simulink subsystem "Controller"  (R2020a)
settings: Solver=VariableStepAuto  StartTime=0.0  StopTime=10.0  RelTol=1e-3
values from neighbouring files (symbols this model uses):
  TMAX = { 32; 32; 32; 32; 32; 32; 32; 32}    [main_adaptive_mpc.m]    (also in matlab.mat = [32 32 32 32 32 32 32 32])
  TMIN = {-26;-26;-26;-26;-26;-26;-26;-26}    [main_adaptive_mpc.m]    (also in matlab.mat = [-26 -26 -26 -26 -26 -26 -26 -26])
  Ts = 0.1    [main_adaptive_mpc.m]    (also in matlab.mat; newNewTraj.m = 0.25; plant_init.m)
  Ui = zeros(1,nU)    [GetAuvSimAndJacobian.m]    (also in main_adaptive_mpc.m = [0;0;0;0;0;0;0;0]; matlab.mat = [0 0 0 0 0 0 0 0])
  Xi = zeros(1,nX)    [GetAuvSimAndJacobian.m]    (also in main_adaptive_mpc.m = [0;0;0;0;0;0;0;0;0;0;0;0]; matlab.mat = [0 0 0 1 0 0 0 0 0 0 0 0 ... (13 elements, 13x1)])
libraries: mpclib x1
settings Model: Creator=Lamarre  LastModifiedBy=Lamarre

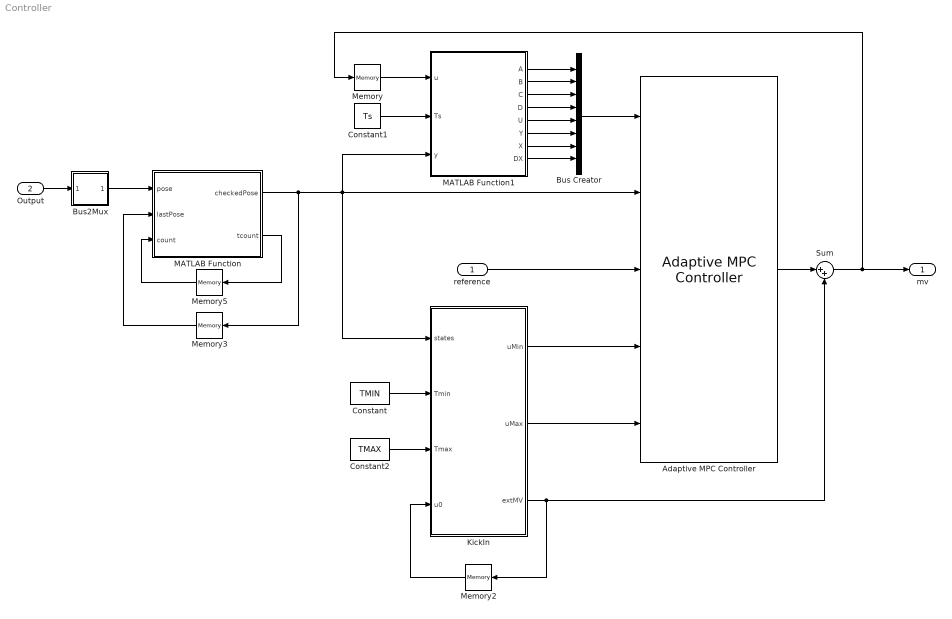
== system Controller ==
  reference : Inport
  Output : Inport  Port=2
  Adaptive MPC Controller : mpclib/Adaptive MPC Controller  SCDEnableBlockLinearizationSpecification=on  mpcobj=mpcobj  enable_value=0  updateMPCinCallerWorkspace=on  md_inport=off  mv_inport=off  uref_inport=off  return_cost=off  return_mvseq=off  return_qpstatus=off  return_xseq=off  return_state=off  return_ovseq=off  state_inport=off  isltv_plant=off  umin_inport=on  umax_inport=on  ymin_inport=off  ymax_inport=off  cc_inport=off  ywt_inport=off  uwt_inport=off  duwt_inport=off  rhoeps_inport=off  pm_inport=off  MaximumP=10  HorizonChoice=FixedHorizon  BlockDataType=double  SampleTimeInherited=off  switch_inport=off
  Bus Creator : BusCreator  Inputs=8
  Bus2Mux : Subsystem
  Constant : Constant  Value=TMIN  VectorParams1D=off
  Constant1 : Constant  Value=Ts
  Constant2 : Constant  Value=TMAX
  KickIn : MATLAB Function  TreatAsAtomicUnit=on  SystemSampleTime=Ts
  MATLAB Function : MATLAB Function  TreatAsAtomicUnit=on
  MATLAB Function1 : MATLAB Function  TreatAsAtomicUnit=on  SystemSampleTime=Ts
  Memory : Memory  InitialCondition=Ui
  Memory2 : Memory  InitialCondition=[0;0;0;0;-7.1;6.94;-7.49;7.65]
  Memory3 : Memory  InitialCondition=Xi
  Memory5 : Memory  InitialCondition=[0,0,0]
  Sum : Sum  Inputs=|++
  mv : Outport
  wires:
  Sum/1 -> mv/1, Memory/1
  Adaptive MPC Controller/1 -> Sum/1
  MATLAB Function1/2(B) -> Bus Creator/2
  MATLAB Function1/1(A) -> Bus Creator/1
  MATLAB Function1/6(Y) -> Bus Creator/6
  MATLAB Function1/8(DX) -> Bus Creator/8
  MATLAB Function1/3(C) -> Bus Creator/3
  MATLAB Function1/4(D) -> Bus Creator/4
  MATLAB Function1/5(U) -> Bus Creator/5
  MATLAB Function1/7(X) -> Bus Creator/7
  Bus Creator/1 -> Adaptive MPC Controller/1
  Memory/1 -> MATLAB Function1/1(u)
  Constant1/1 -> MATLAB Function1/2(Ts)
  KickIn/3(extMV) -> Memory2/1, Sum/2
  Constant2/1 -> KickIn/3(Tmax)
  Memory2/1 -> KickIn/4(u0)
  Constant/1 -> KickIn/2(Tmin)
  KickIn/1(uMin) -> Adaptive MPC Controller/4
  KickIn/2(uMax) -> Adaptive MPC Controller/5
  Output/1 -> Bus2Mux/1(In1)
  Memory5/1 -> MATLAB Function/3(count)
  Memory3/1 -> MATLAB Function/2(lastPose)
  Bus2Mux/1(Out1) -> MATLAB Function/1(pose)
  MATLAB Function/2(tcount) -> Memory5/1
  MATLAB Function/1(checkedPose) -> Memory3/1, MATLAB Function1/3(y), Adaptive MPC Controller/2, KickIn/1(states)
  reference/1 -> Adaptive MPC Controller/3

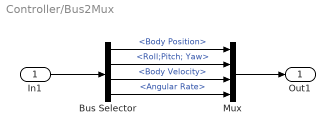
== system Controller/Bus2Mux ==
  In1 : Inport
  Bus Selector : BusSelector  OutputSignals=Body Position,Roll;Pitch; Yaw,Body Velocity,Angular Rate
  Mux : Mux
  Out1 : Outport
  wires:
  Mux/1 -> Out1/1
  In1/1 -> Bus Selector/1
  Bus Selector/2 -> Mux/2  "<Roll;Pitch; Yaw>"
  Bus Selector/4 -> Mux/4  "<Angular Rate>"
  Bus Selector/1 -> Mux/1  "<Body Position>"
  Bus Selector/3 -> Mux/3  "<Body Velocity>"

== matlab function Controller/MATLAB Function1 ==
  data: u input; Ts input; y input; A output; B output; C output; D output; U output; Y output; X output; DX output
function [A,B,C,D,U,Y,X,DX] = TrimPlant(u,Ts,y)
% Lineariser le model dynamique

%x=[y(4:5,1);y(7:12,1)];
%x(5)=x(5)-.85;
[Ac, Bc, Cc, Dc]=AUVStateJacobianFcn(y,u);
% Generate discrete-time model

%  nx = size(Ac,1);
%  nu = size(Bc,2);
%cplant=ss(Ac,Bc,Cc,Dc);
%plant=c2d(cplant,Ts,'zoh');

nx = size(Ac,1);
nu = size(Bc,2);
M = expm([[Ac Bc]*Ts; zeros(nu,nu+nx)]);
A = M(1:nx,1:nx);
B = M(1:nx,nx+1:nx+nu);
C = Cc;
D = Dc;
 %xx=[X(4:5,1);X(7:12)];

% cplant=ss(Ac,Bc,Cc,Dc);
% plant=c2d(cplant,Ts,'zoh');
%plant=ss(A,B,C,D,Ts);

% Nominal conditions for discrete-time plant
U=u.';
Y=(Cc*y + Dc*u).';
X=y.';
DX=(A*y+B*u-y).';

== matlab function Controller/KickIn ==
  data: uMin output; uMax output; states input size=12; Tmin input; Tmax input; extMV output size=8; u0 input size=8
function [uMin,uMax,extMV] = KickIn(states,Tmin,Tmax,u0)

uMin=Tmin;
uMax=Tmax;

% Fonction objective.
fun = @(x)sum(abs(u0.'-x));

% Retrouver la matrice gravité et thruster
Aeq=ThrusterMatrix().';
Beq=Gravity(states).';

% Optimiser la commande pour la condition initial
op=optimoptions('fmincon','Algorithm','sqp');
extMV=-fmincon(fun,u0.',[],[],Aeq,Beq,[],[],[],op).';

% Calculer la nouvelle limite thruster
for i=1:size(extMV,1)
    if extMV(i)>0
        uMax(i)= uMax(i)-extMV(i);
    else
        uMin(i)= uMin(i)-extMV(i);
    end
end

== matlab function Controller/MATLAB Function ==
  data: pose input size=[12 1]; checkedPose output size=[12 1]; lastPose input size=[12 1]; count input size=3; tcount output
function[checkedPose,tcount]= discontinuityCheck(pose,lastPose,count)
           % Cette fonction vérifie et corrige au besoin la discontinuite
           % des angles de rotation.
           tcount=count;
           checkedPose=pose;
           
          for i=4:6 % compute roll pitch yaw
              
              % appliquer la discontinuté actuelle
               if tcount(i-3)>0
                   checkedPose(i)=(pose(i)+pi)+(pi*tcount(i-3));
               elseif tcount<0
                   checkedPose(i)=(pose(i)-pi)+(pi*tcount(i-3));
               end
               
               % calculer la différence entre 2 point
               delta=lastPose(i)-checkedPose(i);
              
               
               % Verifier la discontinuité de laxe
               if abs (delta)>=pi 
                   % Determiner le sens de la discontinuité
                   if delta >0 
                      % Ajouter un tour
                      tcount(i-3)=tcount(i-3)+1;
                      % Recaluler l'angle
                      checkedPose(i)=(pi+pose(i))+(pi*tcount(i-3));
                   else
                      % Soustraire un tour
                      tcount(i-3)=tcount(i-3)-1;
                      % Recaluler l'angle
                      checkedPose(i)=(pose(i)-pi)+(pi*tcount(i-3));
                   end
               end   
           end
